simulink model "b4_1"  (Simulink 7.5)
settings: Solver=ode45  StartTime=0.0  StopTime=10.0  RelTol=1e-3
libraries: commutil2 x10, commdigbbndpm3 x4, commseqgen2 x2, commrandsrc2 x2, commchan3 x1
settings Model: Creator=ADMIN  LastModifiedBy=ADMIN

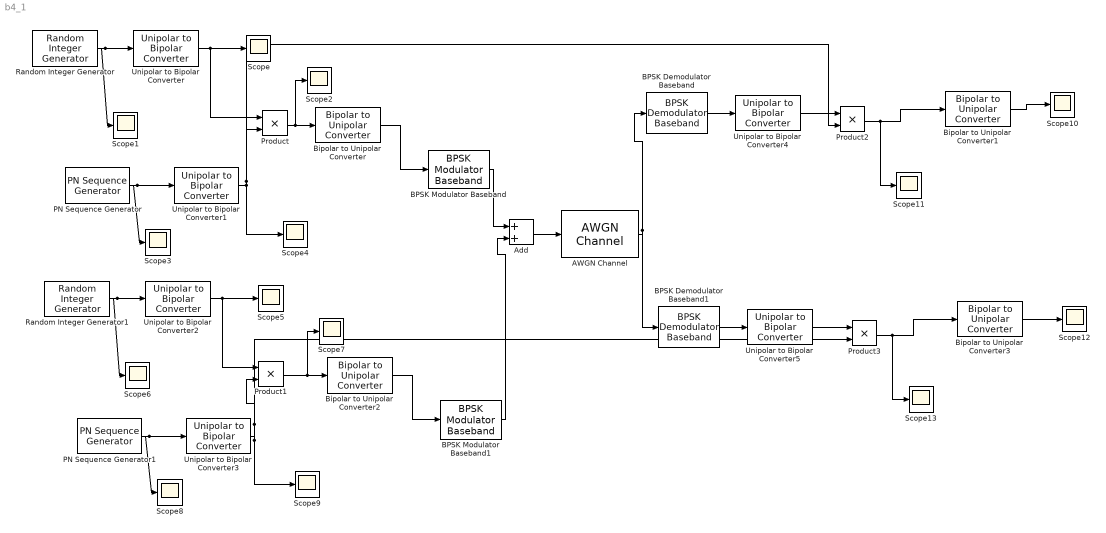
== system b4_1 ==
  AWGN Channel : commchan3/AWGN Channel  SystemSampleTime=-1  seed=67  noiseMode="Signal to noise ratio  (Eb/No)"  EbNodB=10  EsNodB=10  SNRdB=10  bitsPerSym=1  Ps=1  Tsym=1  variance=1
  Add : Sum  OutDataType=fixdt(1, 16)  OutScaling=2^-10
  BPSK Demodulator Baseband : commdigbbndpm3/BPSK Demodulator Baseband  DialogController=commDDGCreate  DialogControllerArgs=DataTag0  Ph=0  DecType=Hard decision  VarSource=Dialog  Variance=1  outDtype=Inherit via internal rule  derotateFactorWordLen=16
  BPSK Demodulator Baseband1 : commdigbbndpm3/BPSK Demodulator Baseband  DialogController=commDDGCreate  DialogControllerArgs=DataTag1  Ph=0  DecType=Hard decision  VarSource=Dialog  Variance=1  outDtype=Inherit via internal rule  derotateFactorWordLen=16
  BPSK Modulator Baseband : commdigbbndpm3/BPSK Modulator Baseband  DialogController=commDDGCreate  DialogControllerArgs=DataTag2  SystemSampleTime=-1  Ph=0  outDtype=single  outWordLen=16  outUDDataType=sfix(16)  outFracLenMode=Best precision  outFracLen=15
  BPSK Modulator Baseband1 : commdigbbndpm3/BPSK Modulator Baseband  DialogController=commDDGCreate  DialogControllerArgs=DataTag3  SystemSampleTime=-1  Ph=0  outDtype=single  outWordLen=16  outUDDataType=sfix(16)  outFracLenMode=Best precision  outFracLen=15
  Bipolar to Unipolar Converter{,1..3} (4 alike) : commutil2/Bipolar to Unipolar Converter  SystemSampleTime=-1  M=2  polarity=Positive  dataType=Same as input
  PN Sequence Generator : commseqgen2/PN Sequence Generator  poly=[1 0 0 0 0 1 1]  ini_sta=[0 0 0 0 0 1]  outBitMaskSource=Dialog parameter  shift=0  Ts=1  frameBased=off  sampPerFrame=1  reset=off  bitPackedOutputs=off  outDataType=double  numPackedBits=8  bitPackDataSigned=off  bitPackedOutDType=double
  PN Sequence Generator1 : commseqgen2/PN Sequence Generator  poly=[1 0 0 0 0 1 1]  ini_sta=[0 0 0 0 0 1]  outBitMaskSource=Dialog parameter  shift=0  Ts=1  frameBased=off  sampPerFrame=1  reset=off  bitPackedOutputs=off  outDataType=double  numPackedBits=8  bitPackDataSigned=off  bitPackedOutDType=double
  Product{,1..3} (4 alike) : Product  OutDataType=fixdt(1, 16)  OutScaling=2^0  RndMeth=Zero
  Random Integer Generator : commrandsrc2/Random Integer Generator  SystemSampleTime=-1  mul=2  seed=0  Ts=1  frameBased=off  sampPerFrame=1  orient=off  outDataType=single
  Random Integer Generator1 : commrandsrc2/Random Integer Generator  SystemSampleTime=-1  mul=2  seed=0  Ts=1  frameBased=off  sampPerFrame=1  orient=off  outDataType=single
  Scope{,1..13} (14 alike) : Scope
      Scope10 settings: SaveName=ScopeData10
      Scope11 settings: SaveName=ScopeData11
      Scope12 settings: SaveName=ScopeData12
      Scope13 settings: SaveName=ScopeData13
      Scope2 settings: SaveName=ScopeData2
      Scope3 settings: SaveName=ScopeData3
      Scope4 settings: SaveName=ScopeData4
      Scope5 settings: SaveName=ScopeData5
      Scope6 settings: SaveName=ScopeData6
      Scope7 settings: SaveName=ScopeData7
      Scope8 settings: SaveName=ScopeData8
      Scope9 settings: SaveName=ScopeData9
  Unipolar to Bipolar Converter{,1..5} (6 alike) : commutil2/Unipolar to Bipolar Converter  SystemSampleTime=-1  M=2  polarity=Positive  dataType=Same as input
  wires:
  Random Integer Generator/1 -> Unipolar to Bipolar Converter/1, Scope1/1
  Unipolar to Bipolar Converter/1 -> Scope/1, Product/1
  PN Sequence Generator/1 -> Unipolar to Bipolar Converter1/1, Scope3/1
  Product/1 -> Bipolar to Unipolar Converter/1, Scope2/1
  Bipolar to Unipolar Converter/1 -> BPSK Modulator Baseband/1
  BPSK Modulator Baseband/1 -> Add/1
  Random Integer Generator1/1 -> Unipolar to Bipolar Converter2/1, Scope6/1
  Unipolar to Bipolar Converter2/1 -> Scope5/1, Product1/1
  PN Sequence Generator1/1 -> Unipolar to Bipolar Converter3/1, Scope8/1
  Unipolar to Bipolar Converter3/1 -> Product1/2, Scope9/1, Product3/2
  Product1/1 -> Bipolar to Unipolar Converter2/1, Scope7/1
  Bipolar to Unipolar Converter2/1 -> BPSK Modulator Baseband1/1
  BPSK Modulator Baseband1/1 -> Add/2
  Add/1 -> AWGN Channel/1
  BPSK Demodulator Baseband/1 -> Unipolar to Bipolar Converter4/1
  Unipolar to Bipolar Converter4/1 -> Product2/1
  Product2/1 -> Bipolar to Unipolar Converter1/1, Scope11/1
  Bipolar to Unipolar Converter1/1 -> Scope10/1
  BPSK Demodulator Baseband1/1 -> Unipolar to Bipolar Converter5/1
  Unipolar to Bipolar Converter5/1 -> Product3/1
  Product3/1 -> Bipolar to Unipolar Converter3/1, Scope13/1
  Bipolar to Unipolar Converter3/1 -> Scope12/1
  AWGN Channel/1 -> BPSK Demodulator Baseband/1, BPSK Demodulator Baseband1/1
  Unipolar to Bipolar Converter1/1 -> Product/2, Scope4/1, Product2/2
